simulink model "mbd_demo"  (R2026a)
settings: Solver=ode45  StopTime=10
settings Model: Creator=Razvan  LastModifiedBy=Razvan

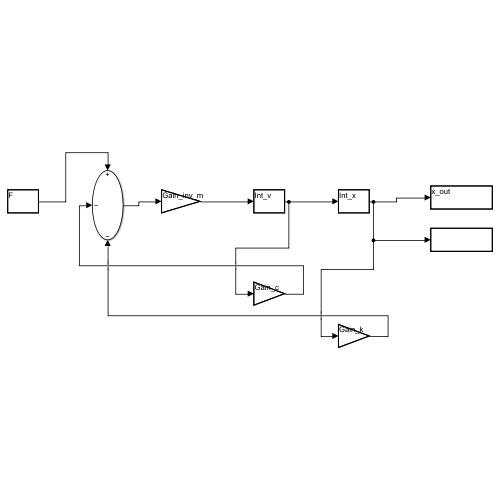
[thumbnail: Simulink's stored preview of the top-level diagram]
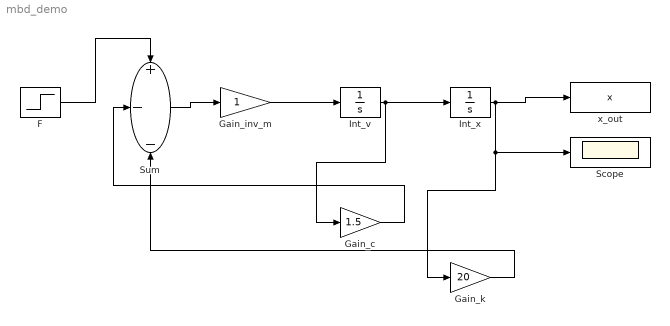
== system mbd_demo ==
  F : Step  Time=0  SampleTime=0
  Gain_c : Gain  Gain=1.5
  Gain_inv_m : Gain
  Gain_k : Gain  Gain=20
  Int_v : Integrator
  Int_x : Integrator
  Scope : Scope
  Sum : Sum  Inputs=+--
  x_out : ToWorkspace  VariableName=x  SampleTime=-1
  wires:
  F/1 -> Sum/1
  Sum/1 -> Gain_inv_m/1
  Gain_inv_m/1 -> Int_v/1
  Int_v/1 -> Int_x/1, Gain_c/1
  Int_x/1 -> Scope/1, Gain_k/1, x_out/1
  Gain_c/1 -> Sum/2
  Gain_k/1 -> Sum/3
